simulink model "batteryDischargeSoln"  (R2015a)
settings: Solver=ode23t  StartTime=0.0  StopTime=1000  RelTol=1e-3  AbsTol=1e-3
undefined symbols (not defined in the file): sigbuilder_block
libraries: fl_lib x9, nesl_utility x4
settings Model: Creator=scastro  LastModifiedBy=sseshadr
settings SimscapeCC: SimscapeLogType=all  SimscapeLogDataHistory=10000

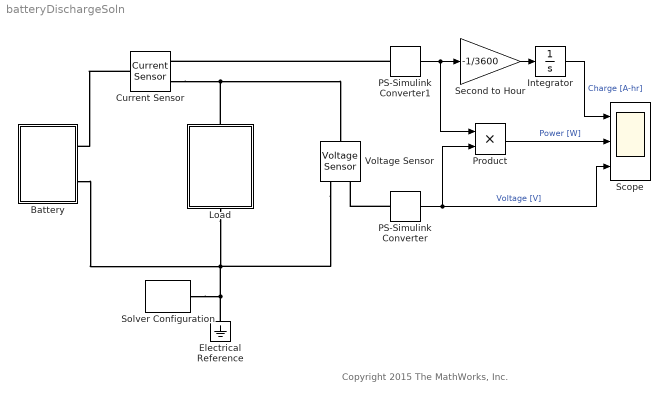
== system batteryDischargeSoln ==
  note: Copyright 2015 The MathWorks, Inc.
  Battery : Subsystem
  Current Sensor : fl_lib/Electrical/Electrical Sensors/Current Sensor
  Electrical Reference : fl_lib/Electrical/Electrical Elements/Electrical Reference
  Integrator : Integrator  InitialCondition=33
  Load : Subsystem
  PS-Simulink Converter : nesl_utility/PS-Simulink Converter  PhysicalDomain=network_engine_domain  SubClassName=ps_output  LeftPortType=input  RightPortType=output  PseudoPeriodic=off  Frequencies=[]  Unit=1  AffineConversion=off
  PS-Simulink Converter1 : nesl_utility/PS-Simulink Converter  PhysicalDomain=network_engine_domain  SubClassName=ps_output  LeftPortType=input  RightPortType=output  PseudoPeriodic=off  Frequencies=[]  Unit=1  AffineConversion=off
  Product : Product
  Scope : Scope  NumInputPorts=3
      settings: TimeRange=1000  YMin=-5~-5~-5  YMax=5~5~5
  Second to Hour : Gain  Gain=-1/3600
  Solver Configuration : nesl_utility/Solver Configuration  PhysicalDomain=network_engine_domain  SubClassName=solver  LeftPortType=input  RightPortType=generic  Accelerate=off  Tones=[]  Harmonics=[]  SimulateNoise=off  Profile=off  UseLocalSampling=off  EnableSwitchedLinearOptims=on  FrequencyDomain=off  UseCCode=off  RelTol=0.001  AbsTol=1e-06  MinStep=1e-09  ToWorkspace=off  RevertToSquareIcSolve=off  NumHomotopyIterations=100  DoDC=off  ResidualTolerance=1e-09  UseLocalSolver=off  LocalSolverChoice=NE_BACKWARD_EULER_ADVANCER  LocalSolverSampleTime=0.001  DoFixedCost=off  MaxNonlinIter=3  MaxModeIter=2  LinearAlgebra=Sparse  DelaysMemoryBudget=1024  AutomaticFiltering=on  FilteringTimeConstant=0.001
  Voltage Sensor : fl_lib/Electrical/Electrical Sensors/Voltage Sensor
  wires:
  PS-Simulink Converter/1 -> Scope/3, Product/2  "Voltage [V]"
  PS-Simulink Converter1/1 -> Second to Hour/1, Product/1
  Integrator/1 -> Scope/1  "Charge [A-hr]"
  Second to Hour/1 -> Integrator/1
  Product/1 -> Scope/2  "Power [W]"
  connections:
  PS-Simulink Converter/LConn1 -- Voltage Sensor/RConn1
  Load/RConn1 -- Current Sensor/RConn2 -- Voltage Sensor/LConn1
  PS-Simulink Converter1/LConn1 -- Current Sensor/RConn1
  Solver Configuration/RConn1 -- Electrical Reference/LConn1 -- Voltage Sensor/RConn2 -- Load/LConn1 -- Battery/RConn2
  Current Sensor/LConn1 -- Battery/RConn1

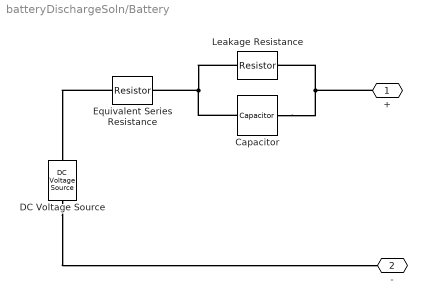
== system batteryDischargeSoln/Battery ==
  Capacitor : fl_lib/Electrical/Electrical Elements/Capacitor  c=5000 F  r=1e-6 Ohm  g=0 1/Ohm  i_specify=off  i_priority=High  i=0 A  v_specify=off  v_priority=High  v=0 V  vc_specify=on  vc_priority=High  vc=0 V
  DC Voltage Source : fl_lib/Electrical/Electrical Sources/DC Voltage Source  v0=100 V
  Equivalent Series Resistance : fl_lib/Electrical/Electrical Elements/Resistor  R=0.01 Ohm  i_specify=off  i_priority=High  i=0 A  v_specify=off  v_priority=High  v=0 V
  Leakage Resistance : fl_lib/Electrical/Electrical Elements/Resistor  R=0.005 Ohm  i_specify=off  i_priority=High  i=0 A  v_specify=off  v_priority=High  v=0 V
  + : PMIOPort  Port=1  Side=Right
  - : PMIOPort  Port=2  Side=Right
  connections:
  Equivalent Series Resistance/LConn1 -- DC Voltage Source/LConn1
  Leakage Resistance/LConn1 -- Capacitor/LConn1 -- Equivalent Series Resistance/RConn1
  Capacitor/RConn1 -- +/RConn1 -- Leakage Resistance/RConn1
  DC Voltage Source/RConn1 -- -/RConn1

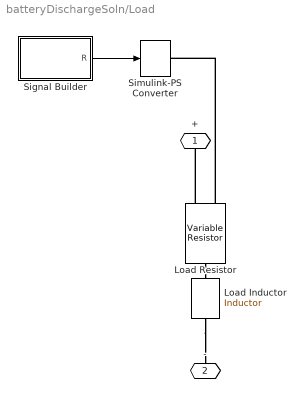
== system batteryDischargeSoln/Load ==
  Load Inductor : fl_lib/Electrical/Electrical Elements/Inductor  l=0.1 H  r=0 Ohm  g=1e-9 1/Ohm  i_specify=off  i_priority=High  i=0 A  v_specify=off  v_priority=High  v=0 V  i_L_specify=off  i_L_priority=High  i_L=0 A
  Load Resistor : fl_lib/Electrical/Electrical Elements/Variable Resistor  Rmin=0 Ohm  i_specify=off  i_priority=High  i=0 A  v_specify=off  v_priority=High  v=0 V
  Signal Builder : Subsystem  Tag=STV Subsys  LoadFcn=sigbuilder_block('load');  StartFcn=sigbuilder_block('start');  StopFcn=sigbuilder_block('stop');  ClipboardFcn=sigbuilder_block('clipboard');  mask(Sigbuilder block){}
      mask help: Simulink:masks:SigbuilderBlock_MD
      mask init:
      | if ~strcmp(get_param(bdroot(gcbh),'SimulationStatus'),'stopped') tuvar = sigbuilder_block('maskInit'); end
      settings: CopyFcn=sigbuilder_block('copy');  DeleteFcn=sigbuilder_block('delete');  ModelCloseFcn=sigbuilder_block('modelClose');  PreSaveFcn=sigbuilder_block('preSave');  PauseFcn=sigbuilder_block('pause');  ContinueFcn=sigbuilder_block('continue');  NameChangeFcn=sigbuilder_block('namechange');  OpenFcn=sigbuilder_block('open',[437.6 199.2 550.4 400 ]);  CloseFcn=sigbuilder_block('close');
      mask Display: plot(0, 0, 100, 100,[2, 2, 32, 32, 2], [68, 8, 8, 68, 68],[32, 2], [38, 38], [32, 19, 2],[53, 60, 44], [32, 17, 17, 2],[16, 16, 31, 31]);txt = getActiveGroup(gcbh);text(2, 100, txt,'verticalAlignment', 'top');
  Simulink-PS Converter : nesl_utility/Simulink-PS Converter  PhysicalDomain=network_engine_domain  SubClassName=ps_input  LeftPortType=input  RightPortType=output  PseudoPeriodic=off  Frequencies=[]  NoiseDistribution=none  NoiseParameters=[]  Unit=Ohm  AffineConversion=off  InputFiltering=off  SimscapeFilterOrder=1  InputFilterTimeConstant=0.001  UdotUserProvided=1
  + : PMIOPort  Port=1  Side=Right
  - : PMIOPort  Port=2  Side=Left
  wires:
  Signal Builder/1(R) -> Simulink-PS Converter/1
  connections:
  Load Resistor/LConn1 -- Simulink-PS Converter/RConn1
  Load Resistor/LConn2 -- +/RConn1
  Load Inductor/RConn1 -- -/RConn1
  Load Resistor/RConn1 -- Load Inductor/LConn1

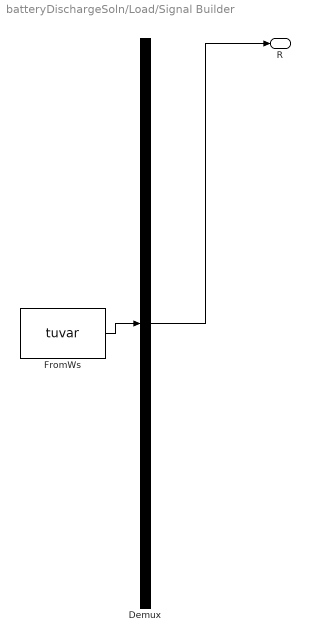
== system batteryDischargeSoln/Load/Signal Builder ==
  Demux : Demux  Tag=STV Demux  Outputs=1
  FromWs : FromWorkspace  Tag=STV FromWs  VariableName=tuvar  SampleTime=0
      SigBuilderData=|
      | common.afterFinalStr = 'Extrapolate'
      | common.sampleTime = 0
      | dataSet.timeRange = [0 1000]
      | dataSet.name = 'Resistance'
      | sbobj.Groups.Name = 'Resistance'
      | sbobj.Groups.Signals.Name = 'R'
      | sbobj.Groups.Signals.XData = [0 100 100 200 200 300 300 400 400 500 500 600 600 700 700 800 800 900 900 1000]
      | sbobj.Groups.Signals.YData = [20 20 5 5 15 15 6 6 20 20 10 10 12 12 2 2 10 10 17 17]
      | sbobj.Groups.TimeRange = [0 1000]
  R : Outport  Tag=STV Outport
  wires:
  Demux/1 -> R/1
  FromWs/1 -> Demux/1
